simulink model "Modele_Lin_BF_C_Avec_Integral"  (R2022a)
settings: Solver=ode45  StartTime=0.0  StopTime=100  RelTol=1e-3  EnableMultiTasking=on
values from neighbouring files (symbols this model uses):
  Jt = 5.8743e-04    (= 0.00058743)    [parametres.m]
  k = 0.0337    [parametres.m]
  Kp = 10/6.28    (= 1.5923566879)    [parametres.m]
  Kv = 0.0497    [parametres.m]
  Kyi = Kci*inv(Ci)    [parametres.m]
  Pente = 8.7060e-10    (= 8.706e-10)    [parametres.m]
  R = 5.8    [parametres.m]
  ro = 1/20    (= 0.05)    [parametres.m]
libraries: simulink x1
settings Model: Creator=reamaa  LastModifiedBy=didouha
settings SolverCC: AlgebraicLoopSolver=TrustRegion
settings DataIOCC: LimitDataPoints=on  SaveFormat=Array  SignalLoggingSaveFormat=ModelDataLogs  ReturnWorkspaceOutputs=off
settings OptimizationCC: BlockReduction=off  BooleanDataType=off  InitFltsAndDblsToZero=on  LifeSpan=inf
settings DebuggingCC: SaveWithParameterizedLinksMsg=none  UnderspecifiedInitializationDetection=Classic  MergeDetectMultiDrivingBlocksExec=none  SignalResolutionControl=TryResolveAllWithWarning  MultiTaskDSMMsg=warning  MultiTaskCondExecSysMsg=none  FcnCallInpInsideContextMsg=warning  UnconnectedInputMsg=warning  UnconnectedOutputMsg=warning  UnconnectedLineMsg=warning  SFUnexpectedBacktrackingDiag=warning  SFNoUnconditionalDefaultTransitionDiag=warning  SFExecutionAtInitializationDiag=none  SFMachineParentedDataDiag=warning  ArithmeticOperatorsInVariantConditions=warning
settings HardwareCC: ProdBitPerPointer=32  ProdBitPerSizeT=32  ProdBitPerPtrDiffT=32  ProdLargestAtomicFloat=None  ProdIntDivRoundTo=Undefined  ProdEndianess=Unspecified  ProdWordSize=32  ProdHWDeviceType=32-bit Generic  TargetUnknown=on
settings ModelReferenceCC: PropagateSignalLabelsOutOfModel=off
settings SFSimCC: SimUseLocalCustomCode=off  CustomCodeUndefinedFunction=UseInterfaceOnly
settings RTWCC: RTWUseLocalCustomCode=off
settings CodeAppCC: StateflowObjectComments=on
settings GRTTargetCC: TargetFcnLib=ansi_tfl_tmw.mat  TargetLangStandard=C89/C90 (ANSI)  CombineOutputUpdateFcns=off  GRTInterface=on
settings ConfigComp: CovMetricSettings=dw  CovSaveCumulativeToWorkspaceVar=on  CovSaveSingleToWorkspaceVar=on  CovExternalEMLEnable=off

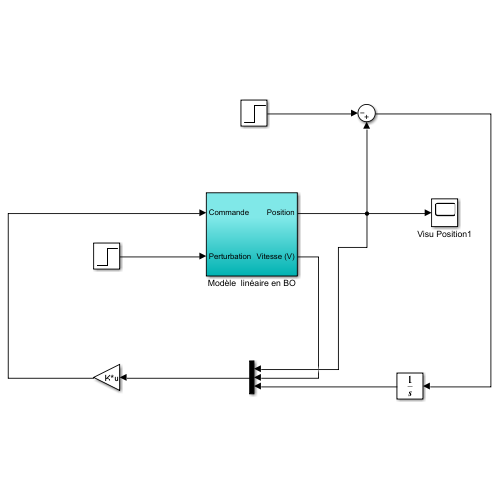
[thumbnail: Simulink's stored preview of the top-level diagram]
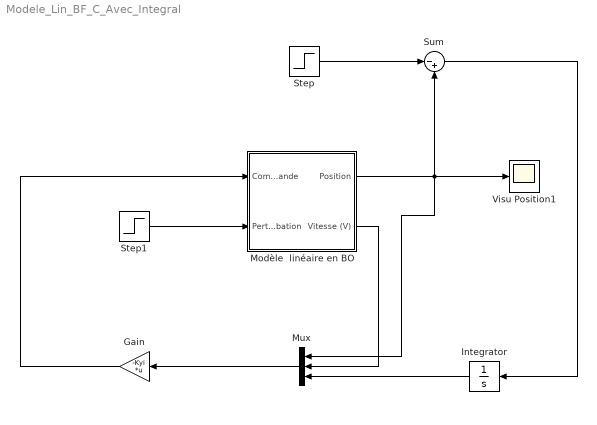
== system Modele_Lin_BF_C_Avec_Integral ==
  Gain : Gain  Gain=-Kyi  Multiplication=Matrix(K*u)
  Integrator : Integrator
  Modèle  linéaire en BO : Subsystem
  Mux : Mux  Inputs=3
  Step : Step  Time=0  SampleTime=0
  Step1 : Step  Time=50  After=0.01  SampleTime=0
  Sum : Sum  Inputs=|-+
  Visu Position1 : Scope
  wires:
  Modèle  linéaire en BO/1(Position) -> Mux/1, Visu Position1/1, Sum/2
  Step/1 -> Sum/1
  Modèle  linéaire en BO/2(Vitesse (V)) -> Mux/2
  Step1/1 -> Modèle  linéaire en BO/2(Perturbation)
  Mux/1 -> Gain/1
  Gain/1 -> Modèle  linéaire en BO/1(Commande)
  Sum/1 -> Integrator/1
  Integrator/1 -> Mux/3

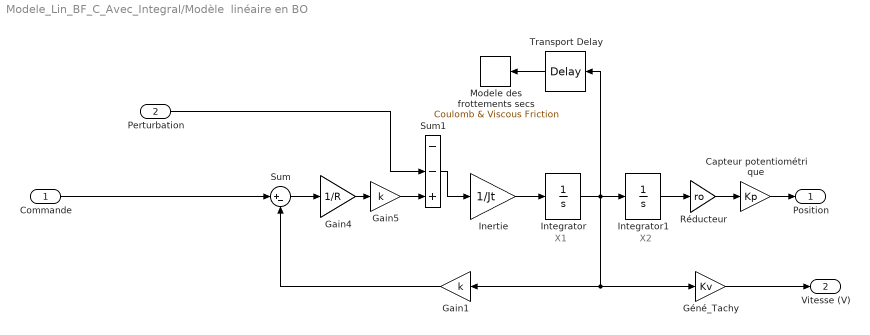
== system Modele_Lin_BF_C_Avec_Integral/Modèle  linéaire en BO ==
  note: X1
  note: X2
  Commande : Inport
  Perturbation : Inport  Port=2
  Capteur potentiométrique : Gain  Gain=Kp  SaturateOnIntegerOverflow=on  OutDataTypeStr=Inherit: Same as input  ParamDataTypeStr=Inherit: Same as input
  Gain1 : Gain  Gain=k  SaturateOnIntegerOverflow=on  OutDataTypeStr=Inherit: Same as input  ParamDataTypeStr=Inherit: Same as input
  Gain4 : Gain  Gain=1/R  SaturateOnIntegerOverflow=on  OutDataTypeStr=Inherit: Same as input  ParamDataTypeStr=Inherit: Same as input
  Gain5 : Gain  Gain=k  SaturateOnIntegerOverflow=on  OutDataTypeStr=Inherit: Same as input  ParamDataTypeStr=Inherit: Same as input
  Géné_Tachy : Gain  Gain=Kv  SaturateOnIntegerOverflow=on  OutDataTypeStr=Inherit: Same as input  ParamDataTypeStr=Inherit: Same as input
  Inertie : Gain  Gain=1/Jt  SaturateOnIntegerOverflow=on  OutDataTypeStr=Inherit: Same as input  ParamDataTypeStr=Inherit: Same as input
  Integrator : Integrator
  Integrator1 : Integrator
  Modele des frottements secs : simulink/Discontinuities/Coulomb & Viscous Friction  offset=Csec  gain=Pente
  Réducteur : Gain  Gain=ro  OutDataTypeStr=Inherit: Same as input  ParamDataTypeStr=Inherit: Same as input
  Sum : Sum  Inputs=|+-  InputSameDT=on  SaturateOnIntegerOverflow=on  OutDataTypeStr=Inherit: Same as first input
  Sum1 : Sum  Inputs=--+  InputSameDT=on  SaturateOnIntegerOverflow=on  OutDataTypeStr=Inherit: Same as first input
  Transport Delay : TransportDelay  DelayTime=0.0001
  Position : Outport
  Vitesse (V) : Outport  Port=2
  wires:
  Géné_Tachy/1 -> Vitesse (V)/1
  Capteur potentiométrique/1 -> Position/1
  Sum1/1 -> Inertie/1
  Réducteur/1 -> Capteur potentiométrique/1
  Integrator1/1 -> Réducteur/1
  Gain1/1 -> Sum/2
  Integrator/1 -> Transport Delay/1, Integrator1/1, Géné_Tachy/1, Gain1/1
  Inertie/1 -> Integrator/1
  Gain4/1 -> Gain5/1
  Sum/1 -> Gain4/1
  Gain5/1 -> Sum1/3
  Perturbation/1 -> Sum1/2
  Commande/1 -> Sum/1
  Transport Delay/1 -> Modele des frottements secs/1
